simulink model "Ground_Z_from_XY"  (R2019a)
settings: Solver=ode45  StartTime=0  StopTime=10  FixedStep=0.002  RelTol=1e-3  AbsTol=1e-6
libraries: Solver_SF x2
settings Model: ExtModeTrigMode=oneshot  ExtModeArmWhenConnect=off  Creator=ywata  LastModifiedBy=msayers
settings SolverCC: AutoScaleAbsTol=off
settings DataIOCC: SaveFormat=Array  SignalLoggingSaveFormat=ModelDataLogs  ReturnWorkspaceOutputs=off  SignalLoggingName=sigsOut
settings OptimizationCC: BlockReduction=off  BooleanDataType=off  LifeSpan=inf
settings DebuggingCC: SaveWithParameterizedLinksMsg=none  UnderspecifiedInitializationDetection=Classic  MergeDetectMultiDrivingBlocksExec=none  SignalResolutionControl=TryResolveAllWithWarning  MultiTaskDSMMsg=warning  MultiTaskCondExecSysMsg=none  FcnCallInpInsideContextMsg=warning  StateNameClashWarn=warning  SFUnexpectedBacktrackingDiag=warning  SFNoUnconditionalDefaultTransitionDiag=warning  ArithmeticOperatorsInVariantConditions=warning
settings HardwareCC: ProdBitPerPointer=32  ProdBitPerSizeT=32  ProdBitPerPtrDiffT=32  ProdLargestAtomicFloat=None  ProdIntDivRoundTo=Undefined  ProdEndianess=Unspecified  ProdWordSize=32  ProdHWDeviceType=32-bit Generic  TargetUnknown=on
settings ModelReferenceCC: PropagateSignalLabelsOutOfModel=off
settings SFSimCC: SimUseLocalCustomCode=off
settings RTWCC: TemplateMakefile=grt_vc.tmf  RTWUseLocalCustomCode=off
settings CodeAppCC: StateflowObjectComments=on
settings GRTTargetCC: TargetFcnLib=ansi_tfl_tmw.mat  TargetLangStandard=C89/C90 (ANSI)  CombineOutputUpdateFcns=off  GRTInterface=on
settings ConfigComp: CovMetricSettings=dw  CovSaveCumulativeToWorkspaceVar=on  CovSaveSingleToWorkspaceVar=on  CovExternalEMLEnable=off  CovSFcnEnable=off

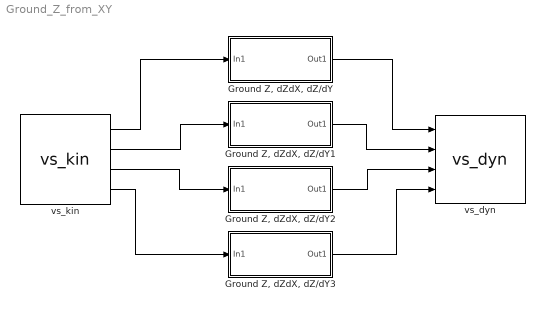
== system Ground_Z_from_XY ==
  "Ground Z, dZdX, dZ/dY" : Subsystem
  "Ground Z, dZdX, dZ/dY1" : Subsystem
  "Ground Z, dZdX, dZ/dY2" : Subsystem
  "Ground Z, dZdX, dZ/dY3" : Subsystem
  vs_dyn : Solver_SF/CarSim Multi-Wrappers/vs_dyn  Priority=4  SIMFILE=simfile.sim
  vs_kin : Solver_SF/CarSim Multi-Wrappers/vs_kin  Priority=3  SIMFILE=simfile.sim
  wires:
  vs_kin/1 -> "Ground Z, dZdX, dZ/dY"/1(In1)
  "Ground Z, dZdX, dZ/dY1"/1(Out1) -> vs_dyn/2
  vs_kin/3 -> "Ground Z, dZdX, dZ/dY2"/1(In1)
  "Ground Z, dZdX, dZ/dY2"/1(Out1) -> vs_dyn/3
  "Ground Z, dZdX, dZ/dY3"/1(Out1) -> vs_dyn/4
  vs_kin/4 -> "Ground Z, dZdX, dZ/dY3"/1(In1)
  vs_kin/2 -> "Ground Z, dZdX, dZ/dY1"/1(In1)
  "Ground Z, dZdX, dZ/dY"/1(Out1) -> vs_dyn/1

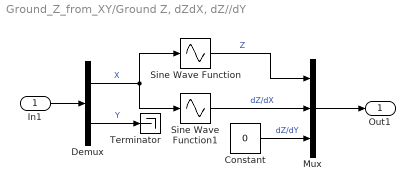
== system Ground_Z_from_XY/Ground Z, dZdX, dZ//dY ==
  In1 : Inport  PortDimensions=2
  Constant : Constant  Value=0
  Demux : Demux  Outputs=2
  Mux : Mux  Inputs=3
  Sine Wave Function : Sin  TimeSource=Use external signal  Bias=1  Frequency=2*pi/100  SampleTime=0
  Sine Wave Function1 : Sin  TimeSource=Use external signal  Amplitude=2*pi/100  Frequency=2*pi/100  Phase=pi/2  SampleTime=0
  Terminator : Terminator
  Out1 : Outport  PortDimensions=3
  wires:
  Sine Wave Function1/1 -> Mux/2  "dZ/dX"
  Demux/2 -> Terminator/1  "Y"
  Sine Wave Function/1 -> Mux/1  "Z"
  Constant/1 -> Mux/3  "dZ/dY"
  Mux/1 -> Out1/1
  Demux/1 -> Sine Wave Function1/1, Sine Wave Function/1  "X"
  In1/1 -> Demux/1

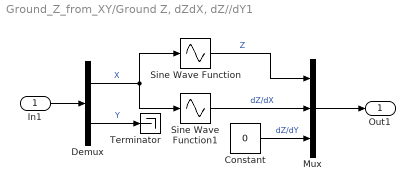
== system Ground_Z_from_XY/Ground Z, dZdX, dZ//dY1 ==
  In1 : Inport  PortDimensions=2
  Constant : Constant  Value=0
  Demux : Demux  Outputs=2
  Mux : Mux  Inputs=3
  Sine Wave Function : Sin  TimeSource=Use external signal  Bias=1  Frequency=2*pi/100  SampleTime=0
  Sine Wave Function1 : Sin  TimeSource=Use external signal  Amplitude=2*pi/100  Frequency=2*pi/100  Phase=pi/2  SampleTime=0
  Terminator : Terminator
  Out1 : Outport  PortDimensions=3
  wires:
  Sine Wave Function1/1 -> Mux/2  "dZ/dX"
  Demux/2 -> Terminator/1  "Y"
  Sine Wave Function/1 -> Mux/1  "Z"
  Constant/1 -> Mux/3  "dZ/dY"
  Mux/1 -> Out1/1
  Demux/1 -> Sine Wave Function1/1, Sine Wave Function/1  "X"
  In1/1 -> Demux/1

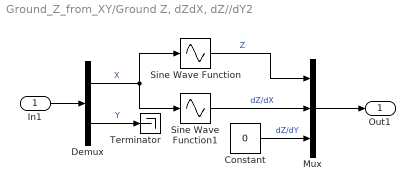
== system Ground_Z_from_XY/Ground Z, dZdX, dZ//dY2 ==
  In1 : Inport  PortDimensions=2
  Constant : Constant  Value=0
  Demux : Demux  Outputs=2
  Mux : Mux  Inputs=3
  Sine Wave Function : Sin  TimeSource=Use external signal  Bias=1  Frequency=2*pi/100  SampleTime=0
  Sine Wave Function1 : Sin  TimeSource=Use external signal  Amplitude=2*pi/100  Frequency=2*pi/100  Phase=pi/2  SampleTime=0
  Terminator : Terminator
  Out1 : Outport  PortDimensions=3
  wires:
  In1/1 -> Demux/1
  Mux/1 -> Out1/1
  Demux/2 -> Terminator/1  "Y"
  Constant/1 -> Mux/3  "dZ/dY"
  Sine Wave Function1/1 -> Mux/2  "dZ/dX"
  Demux/1 -> Sine Wave Function1/1, Sine Wave Function/1  "X"
  Sine Wave Function/1 -> Mux/1  "Z"

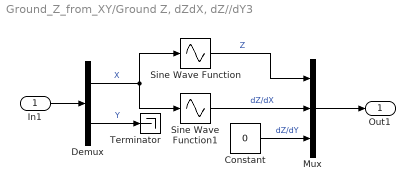
== system Ground_Z_from_XY/Ground Z, dZdX, dZ//dY3 ==
  In1 : Inport  PortDimensions=2
  Constant : Constant  Value=0
  Demux : Demux  Outputs=2
  Mux : Mux  Inputs=3
  Sine Wave Function : Sin  TimeSource=Use external signal  Bias=1  Frequency=2*pi/100  SampleTime=0
  Sine Wave Function1 : Sin  TimeSource=Use external signal  Amplitude=2*pi/100  Frequency=2*pi/100  Phase=pi/2  SampleTime=0
  Terminator : Terminator
  Out1 : Outport  PortDimensions=3
  wires:
  Sine Wave Function1/1 -> Mux/2  "dZ/dX"
  Demux/2 -> Terminator/1  "Y"
  Sine Wave Function/1 -> Mux/1  "Z"
  Constant/1 -> Mux/3  "dZ/dY"
  Mux/1 -> Out1/1
  Demux/1 -> Sine Wave Function1/1, Sine Wave Function/1  "X"
  In1/1 -> Demux/1
